simulink model "MIL4L3_SW6_V1_20220211"  (R2018b)
settings: Solver=FixedStepAuto  StartTime=0.0  StopTime=inf  FixedStep=0.001  RelTol=1e-3
PreLoadFcn:
  | A0_MILtest;
undefined symbols (not defined in the file or in its folder): Clb_ICADirect_LaneDisp_StateFive, Clb_ICADirect_LaneDisp_StateFour, Clb_ICADirect_LaneDisp_StateOne, Clb_ICADirect_LaneDisp_StateThree, Clb_ICADirect_LaneDisp_StateTwo, Clb_ICADirect_LaneDisp_StateZero, Clb_ICADirect_LaneDispSW, Clb_ICADirect_TrnLghtsCom_Switch, Clb_ICADirect_TrnLghtsCom_Value, Clb_ICADirect_TrnLghtsCrtl_Inhb, IMAP_Clb_ACU_Driver_Belt, IMAP_Clb_ACU_Driver_Belt_Over, IMAP_Clb_ACU_Passenger_Belt, IMAP_Clb_ACU_Passenger_Belt_Over, IMAP_Clb_ACU_RearLeft_Belt, IMAP_Clb_ACU_RearLeft_Belt_Over, IMAP_Clb_ACU_RearMiddle_Belt, IMAP_Clb_ACU_RearMiddle_Belt_Over, IMAP_Clb_ACU_RearRight_Belt, IMAP_Clb_ACU_RearRight_Belt_Over, IMAP_Clb_AEB_Switch, IMAP_Clb_AEB_Switch_Over, IMAP_Clb_ALC_TLC_Mode, IMAP_Clb_ALC_TLC_Mode_Over, IMAP_Clb_BCM_Battery_Voltage, IMAP_Clb_BCM_Battery_Voltage_Over, IMAP_Clb_BCM_BrakeLamp_State, IMAP_Clb_BCM_BrakeLamp_State_Over, IMAP_Clb_BCM_CHMSL_Status, IMAP_Clb_BCM_CHMSL_Status_Over, IMAP_Clb_BCM_Door_Lock_State, IMAP_Clb_BCM_Door_Lock_State_Over, IMAP_Clb_BCM_FrontWiper_State, IMAP_Clb_BCM_FrontWiper_State_Over, IMAP_Clb_BCM_FrontWiper_Switch, IMAP_Clb_BCM_FrontWiper_Switch_Over, IMAP_Clb_BCM_HazardLamp, IMAP_Clb_BCM_HazardLamp_Over, IMAP_Clb_BCM_HazardLamp_Switch, IMAP_Clb_BCM_HazardLamp_Switch_Over, IMAP_Clb_BCM_HighBeam_State, IMAP_Clb_BCM_HighBeam_State_Over, IMAP_Clb_BCM_Ignition_State, IMAP_Clb_BCM_Ignition_State_Over, IMAP_Clb_BCM_IHBC_Enabled, IMAP_Clb_BCM_IHBC_Enabled_Over, IMAP_Clb_BCM_Left_Light, IMAP_Clb_BCM_Left_Light_Over, IMAP_Clb_BCM_LeftTurn_Switch, IMAP_Clb_BCM_LeftTurn_Switch_Over, IMAP_Clb_BCM_LF_Door_State, IMAP_Clb_BCM_LF_Door_State_Over, IMAP_Clb_BCM_LowBeam_State, IMAP_Clb_BCM_LowBeam_State_Over, IMAP_Clb_BCM_LR_Door_State, IMAP_Clb_BCM_LR_Door_State_Over, IMAP_Clb_BCM_RF_Door_State, IMAP_Clb_BCM_RF_Door_State_Over, IMAP_Clb_BCM_Right_Light, IMAP_Clb_BCM_Right_Light_Over ... (+547)
libraries: CarMaker4SL x2153, simulink x292, dspstat3 x3, canmsglib x2, simulink_extras x1
(part 10 of 52)

== system MIL4L3_SW6_V1_20220211/CarMaker/VehicleControl/Function/ICA ==
  note: ICAB
  note: 状态机
  note: ICA模式：
      | 0 Unactive，1 LF，2 LF(SingleLane)，3 VF，4 LC
  note: ICA状态：
      | 0 sysOFF，1 inhibit，2 ready，3 normal，4 degradation
      | 5 fault，6 active，7 sysON，8 systoON
  Bus Selector2 : BusSelector  OutputSignals=IMAPve_g_EPS_SW_Trq,IMAPve_d_EPS_Trq_State,IMAPve_d_SAS_Clb_State,IMAPve_d_SAS_Trim_State,IMAPve_d_EPS_TrqLim_State,IMAPve_g_ESC_LatAcc,IMAPve_d_ESC_LatAcc_Valid,IMAPve_g_ESC_YawRate,IMAPve_d_ESC_YawRate_Valid,IMAPve_g_ESC_VehSpd,IMAPve_g_ESC_LonAcc,IMAPve_d_ESC_LonAcc_Valid,IMAPve_g_ESC_DySlope_Accuracy,IMAPve_g_ESC_DySlope,IMAPve_g_SW_Angle,IMAPve_g_SW_Angle_Speed,IMAPve_d_BCM_HazardLamp,IMAPve_d_BCM_Left_Light,IMAPve_d_BCM_Right_Light,IMAPve_d_BCM_Opening_State,IMAPve_d_SCC_Left_SwitchSig,IMAPve_g_EMS_RealPedal,IMAPve_d_EMS_AccPedal_Fault,IMAPve_d_ESC_Veh_Standstill,IMAPve_d_TCU_Actual_Gear,IMAPve_d_ACU_Driver_Belt,IMAPve_d_SWS_Failure_Status,IMAPve_d_ESC_ESC_Active,IMAPve_d_ESC_TCS_Active,IMAPve_d_ESC_VehSpd_Valid,IMAPve_d_ESC_ABS_Active,IMAPve_d_TCU_Select_ATMode,IMAPve_d_BCM_FrontWiper_State,IMAPve_d_ACU_Passenger_Belt,IMAPve_d_EMS_Brake_Pedal,IMAPve_d_BCM_LowBeam_State,IMAPve_d_BCM_HighBeam_State,IMAPve_d_EPS_Steer_Hold_State,IMAPve_d_EPS_Warning_State,IMAPve_d_ESC_AVH_Status,IMAPve_g_ORI_L0_C3,IMAPve_g_ORI_L0_C2,IMAPve_g_ORI_L0_C1,IMAPve_g_ORI_L0_C0,IMAPve_d_ORI_L0_Type,IMAPve_g_ORI_L0_VR,IMAPve_g_ORI_L0_W,IMAPve_g_ORI_L1_C3,IMAPve_g_ORI_L1_C2,IMAPve_g_ORI_L1_C1,IMAPve_g_ORI_L1_C0,IMAPve_d_ORI_L1_Type,IMAPve_g_ORI_L1_VR,IMAPve_g_ORI_L1_W,IMAPve_g_ORI_R0_C3,IMAPve_g_ORI_R0_C2,IMAPve_g_ORI_R0_C1,IMAPve_g_ORI_R0_C0,IMAPve_d_ORI_R0_LT,IMAPve_g_ORI_R0_VR,IMAPve_g_ORI_R0_W,IMAPve_g_ORI_R1_C3,IMAPve_g_ORI_R1_C2,IMAPve_g_ORI_R1_C1,IMAPve_g_ORI_R1_C0,IMAPve_d_ORI_R1_LT,IMAPve_g_ORI_R1_VR,IMAPve_g_ORI_R1_W,IMAPve_d_Fusion_Status,IMAPve_d_obj_Num,IMAPva_d_obj_id,IMAPva_g_obj_pos_x,IMAPva_g_obj_pos_y,IMAPva_g_obj_vel_x,IMAPva_g_obj_vel_y,IMAPva_g_obj_acc_x,IMAPva_g_obj_acc_y,IMAPva_g_obj_pos_var_x,IMAPva_g_obj_pos_var_y,IMAPva_g_obj_pos_var_xy,IMAPva_g_obj_width,IMAPva_g_obj_length,IMAPva_d_obj_class,IMAPva_d_obj_lane,IMAPva_d_obj_status,IMAPva_d_obj_age,IMAPva_d_obj_TurnLight,IMAPva_d_obj_BrakeLight,IMAPva_d_obj_MotionStatus,IMAPve_d_Road_Type,IMAPve_g_L0_C0,IMAPve_g_L0_C1,IMAPve_g_L0_C2,IMAPve_g_L0_C3,IMAPve_g_L0_VR,IMAPve_d_L0_Q,IMAPve_d_L0_Type,IMAPve_g_L0_W,IMAPve_g_R0_C0,IMAPve_g_R0_C1,IMAPve_g_R0_C2,IMAPve_g_R0_C3,IMAPve_g_R0_VR,IMAPve_d_R0_Q,IMAPve_d_R0_Type,IMAPve_g_R0_W,IMAPve_g_L1_C0,IMAPve_g_L1_C1,IMAPve_g_L1_C2,IMAPve_g_L1_C3,IMAPve_g_L1_VR,IMAPve_d_L1_Q,IMAPve_d_L1_Type,IMAPve_g_L1_W,IMAPve_g_R1_C0,IMAPve_g_R1_C1,IMAPve_g_R1_C2,IMAPve_g_R1_C3,IMAPve_g_R1_VR,IMAPve_d_R1_Q,IMAPve_d_R1_Type,IMAPve_g_R1_W,IMAPve_g_L0_C0_Back,IMAPve_g_L0_C1_Back,IMAPve_g_L0_C2_Back,IMAPve_g_L0_C3_Back,IMAPve_g_L0_Range_Back,IMAPve_g_R0_C0_Back,IMAPve_g_R0_C1_Back,IMAPve_g_R0_C2_Back,IMAPve_g_R0_C3_Back,IMAPve_g_R0_Range_Back,IMAPve_g_L1_C0_Back,IMAPve_g_L1_C1_Back,IMAPve_g_L1_C2_Back,IMAPve_g_L1_C3_Back,IMAPve_g_L1_Range_Back,IMAPve_g_R1_C0_Back,IMAPve_g_R1_C1_Back,IMAPve_g_R1_C2_Back,IMAPve_g_R1_C3_Back,IMAPve_g_R1_Range_Back,IMAPve_d_APA_AutoPark_WorkSt
  Bus Selector3 : BusSelector  OutputSignals=IMAPve_d_BCM_HazardLamp_Switch,IMAPve_d_BCM_LeftTurn_Switch,IMAPve_d_BCM_RightTurn_Switch,IMAPve_g_Lrg_C0_BACK,IMAPve_g_Lrg_C1_BACK,IMAPve_g_Lrg_C2_BACK,IMAPve_g_Lrg_C3_BACK,IMAPve_g_Lrg_VR_Start_BACK,IMAPve_g_Lrg_VR_End_BACK,IMAPve_d_Lrg_Q_BACK,IMAPve_d_Lrg_TYPE_BACK,IMAPve_g_Rrg_C0_BACK,IMAPve_g_Rrg_C1_BACK,IMAPve_g_Rrg_C2_BACK,IMAPve_g_Rrg_C3_BACK,IMAPve_g_Rrg_VR_Start_BACK,IMAPve_g_Rrg_VR_End_BACK,IMAPve_d_Rrg_Q_BACK,IMAPve_d_Rrg_TYPE_BACK
  Bus Selector : BusSelector  OutputSignals=FDMMve_d_IcaFcnConf,FDMMve_d_SignalTStamp
  Bus Selector1 : BusSelector  OutputSignals=ICABve_d_ICAMode
  BusCreator : BusCreator  Inputs=16
  Clock : Clock
  Compare To Constant : simulink/Logic and Bit Operations/Compare To Constant  relop===  const=4  OutDataTypeStr=boolean
  Constant : Constant  Value=0  OutDataTypeStr=uint32
  Constant1 : Constant  Value=0  OutDataTypeStr=uint32
  Constant2 : Constant  Value=0  OutDataTypeStr=uint16
  Constant3 : Constant  OutDataTypeStr=uint8
  Constant4 : Constant  Value=0  OutDataTypeStr=uint8
  Constant5 : Constant  OutDataTypeStr=uint8
  Constant6 : Constant  Value=0  OutDataTypeStr=uint8
  Data Type  Conversion : DataTypeConversion
  Data Type  Conversion1 : DataTypeConversion
  Data Type Conversion{,3..7,45,94,115..116} (10 alike) : DataTypeConversion
  Data Type Conversion1 : DataTypeConversion  OutDataTypeStr=uint16
  Data Type Conversion2 : DataTypeConversion  OutDataTypeStr=uint16
  Define CM Dict : CarMaker4SL/Define CM Dict  xname=User.IO.Out.VR_RR  xmono=off  xtype=Double4  xdvaplace=IO_Out  xnstates=0  xfirststate=0  xinitial=50
  Define CM Dict1 : CarMaker4SL/Define CM Dict  xname=User.IO.In.LineChangeFlag  xmono=off  xtype=Double4  xdvaplace=VC  xnstates=0  xfirststate=0  xinitial=0
  Define CM Dict2 : CarMaker4SL/Define CM Dict  xname=User.IO.In.ICABState  xmono=off  xtype=Double4  xdvaplace=VC  xnstates=0  xfirststate=0  xinitial=0
  Define CM Dict26 : CarMaker4SL/Define CM Dict  xname=User.IO.In.ICABve_g_SteerAngleCmd  xmono=off  xtype=Double4  xdvaplace=VC  xnstates=0  xfirststate=0  xinitial=0
  Define CM Dict3 : CarMaker4SL/Define CM Dict  xname=User.IO.Out.VR_R  xmono=off  xtype=Double4  xdvaplace=IO_Out  xnstates=0  xfirststate=0  xinitial=50
  Define CM Dict4 : CarMaker4SL/Define CM Dict  xname=User.IO.Out.VR_LL  xmono=off  xtype=Double4  xdvaplace=IO_Out  xnstates=0  xfirststate=0  xinitial=50
  Define CM Dict5 : CarMaker4SL/Define CM Dict  xname=User.IO.Out.VR_L  xmono=off  xtype=Double4  xdvaplace=IO_Out  xnstates=0  xfirststate=0  xinitial=50
  Define CM Dict6 : CarMaker4SL/Define CM Dict  xname=User.IO.Out.stLCRMode  xmono=off  xtype=Double4  xdvaplace=IO_Out  xnstates=0  xfirststate=0  xinitial=0
  Demux : Demux  Outputs=20
  EPS Position Control Enable Management (EPSPCEM)_KDK1 : Subsystem
  EPS_State_Mashine : Subsystem
  Enabled Subsystem : Subsystem  TreatAsAtomicUnit=on
  Goto1 : Goto  Commented=on  GotoTag=ICAS_output  TagVisibility=global
  ICAB : ModelReference  ModelNameDialog=ICAB_V51_G59_SW6_0127_MIL.slxp  ModelReferenceVersion=1.2185  CopyOfModelProtected=on
  Memory : Memory
  Read CM Dict : CarMaker4SL/Read CM Dict  xname=User.IO.Out.VR_RR  xsync=off
  Read CM Dict1 : CarMaker4SL/Read CM Dict  xname=User.IO.Out.VR_R  xsync=off
  Read CM Dict2 : CarMaker4SL/Read CM Dict  xname=User.IO.Out.VR_LL  xsync=off
  Read CM Dict3 : CarMaker4SL/Read CM Dict  xname=User.IO.Out.VR_L  xsync=off
  Switch{,1..3} (4 alike) : Switch  Threshold=20
  Write CM Dict : CarMaker4SL/Write CM Dict  xname=User.IO.Out.stLCRMode  xsync=off
  Write CM Dict1 : CarMaker4SL/Write CM Dict  xname=User.IO.In.LineChangeFlag  xsync=off
  Write CM Dict17 : CarMaker4SL/Write CM Dict  xname=User.IO.In.ICABve_g_SteerAngleCmd  xsync=off
  Write CM Dict2 : CarMaker4SL/Write CM Dict  xname=User.IO.In.ICABState  xsync=off
  ICAS_output : Outport
  tag scope: EPS_LKA_State_ica=global, ICAB_output=global, ICABva_d_ICAB2ACCS=global, ICABve_d_ICAState=global, ICAMode=global
  wires:
  [FDMM_output] -> Bus Selector/1  "FDMM_output"
  ICAB/2 -> BusCreator/2  "ICABve_d_SignalTStamp"
  Data Type Conversion2/1 -> [EPS_LKA_State_ica], EPS Position Control Enable Management (EPSPCEM)_KDK1/2(EPS_Ctr_State)
  EPS_State_Mashine/1(EPS_Ctr_State) -> Memory/1
  Data Type Conversion1/1 -> EPS_State_Mashine/1(EPS_CMD_KDK)
  EPS Position Control Enable Management (EPSPCEM)_KDK1/1(stEPS_State_Ctl_CMD) -> Data Type Conversion1/1  "EPS_State_Ctl"
  Bus Selector1/1 -> EPS Position Control Enable Management (EPSPCEM)_KDK1/1(EPSPCEM__bsTHState)  "<ICABve_d_ICAMode>"
  Bus Selector/1 -> Data Type Conversion/1  "<FDMMve_d_IcaFcnConf>"
  Clock/1 -> Data Type Conversion94/1
  [ACCSva_d_ACCS2ICAB] -> ICAB/2  "ACCSva_d_ACCS2ICA"
  ? -> Goto1/1, ICAS_output/1
  Data Type Conversion94/1 -> ICAB/1  "System_Clock"
  BusCreator/1 -> Bus Selector1/1, [ICAB_output]
  Data Type  Conversion/1 -> Data Type  Conversion1/1, BusCreator/4  "ICABve_g_SteerAngleCmd"
  Data Type Conversion116/1 -> Write CM Dict2/1
  [IMAP_Output] -> Bus Selector3/1, Bus Selector2/1  "FDMM_output"
  [EPS_LKA_State_ica] -> ICAB/5
  ICAB/16 -> BusCreator/16  "ICABve_g_ob011L_100"
  ICAB/15 -> BusCreator/15  "ICABve_g_ob011H_100"
  ICAB/14 -> BusCreator/14  "ICABve_g_ob010L_100"
  ICAB/13 -> BusCreator/13  "ICABve_g_ob010H_100"
  ICAB/12 -> BusCreator/12  "ICABve_g_ob8L_10"
  ICAB/11 -> BusCreator/11  "ICABve_g_ob8H_10"
  Bus Selector/2 -> ICAB/4  "<FDMMve_d_SignalTStamp>"
  Data Type  Conversion1/1 -> Write CM Dict17/1  "ICABve_g_SteerAngleCmd"
  Data Type Conversion45/1 -> Write CM Dict1/1
  Enabled Subsystem/1(Out1) -> Data Type Conversion45/1
  Compare To Constant/1 -> Enabled Subsystem/Enable
  ICAB/1 -> [ICABva_d_ICAB2ACCS], BusCreator/1  "ICABva_d_ICAB2ACCS"
  ICAB/4 -> Data Type  Conversion/1
  Data Type Conversion115/1 -> [ICAMode], BusCreator/5  "ICABve_d_ICAMode"
  ICAB/6 -> [ICABve_d_ICAState], BusCreator/6, Data Type Conversion116/1  "ICABve_d_ICAState"
  ICAB/7 -> BusCreator/7  "ICABve_d_LKATorqueReq"
  ICAB/8 -> BusCreator/8  "ICABve_g_LKATorqueReq_Value"
  ICAB/9 -> BusCreator/9  "ICABve_g_ob7H_10"
  ICAB/10 -> BusCreator/10  "ICABve_g_ob7L_10"
  Demux/16 -> Data Type Conversion7/1
  ICAB/3 -> BusCreator/3, Demux/1  "ICABva_d_ICAB2HMI"
  Data Type Conversion7/1 -> Write CM Dict/1  "stLCRMode"
  Memory/1 -> Data Type Conversion2/1
  Data Type Conversion/1 -> ICAB/3
  Bus Selector2/118 -> ICAB/123  "<IMAPve_g_R1_C3>"
  Bus Selector2/120 -> ICAB/125  "<IMAPve_d_R1_Q>"
  Bus Selector2/117 -> ICAB/122  "<IMAPve_g_R1_C2>"
  Bus Selector2/121 -> ICAB/126  "<IMAPve_d_R1_Type>"
  Bus Selector2/116 -> ICAB/121  "<IMAPve_g_R1_C1>"
  Bus Selector2/122 -> ICAB/127  "<IMAPve_g_R1_W>"
  Bus Selector2/115 -> ICAB/120  "<IMAPve_g_R1_C0>"
  Bus Selector2/123 -> ICAB/128  "<IMAPve_g_L0_C0_Back>"
  Bus Selector2/114 -> ICAB/119  "<IMAPve_g_L1_W>"
  Bus Selector2/124 -> ICAB/129  "<IMAPve_g_L0_C1_Back>"
  Bus Selector2/113 -> ICAB/118  "<IMAPve_d_L1_Type>"
  Bus Selector2/125 -> ICAB/130  "<IMAPve_g_L0_C2_Back>"
  Bus Selector2/112 -> ICAB/117  "<IMAPve_d_L1_Q>"
  Bus Selector2/126 -> ICAB/131  "<IMAPve_g_L0_C3_Back>"
  Bus Selector2/127 -> ICAB/132  "<IMAPve_g_L0_Range_Back>"
  Bus Selector2/110 -> ICAB/115  "<IMAPve_g_L1_C3>"
  Bus Selector2/128 -> ICAB/133  "<IMAPve_g_R0_C0_Back>"
  Bus Selector2/109 -> ICAB/114  "<IMAPve_g_L1_C2>"
  Bus Selector2/129 -> ICAB/134  "<IMAPve_g_R0_C1_Back>"
  Bus Selector2/108 -> ICAB/113  "<IMAPve_g_L1_C1>"
  Bus Selector2/130 -> ICAB/135  "<IMAPve_g_R0_C2_Back>"
  Bus Selector2/107 -> ICAB/112  "<IMAPve_g_L1_C0>"
  Bus Selector2/131 -> ICAB/136  "<IMAPve_g_R0_C3_Back>"
  Bus Selector2/106 -> ICAB/111  "<IMAPve_g_R0_W>"
  Bus Selector2/132 -> ICAB/137  "<IMAPve_g_R0_Range_Back>"
  Bus Selector2/105 -> ICAB/110  "<IMAPve_d_R0_Type>"
  Bus Selector2/133 -> ICAB/138  "<IMAPve_g_L1_C0_Back>"
  Bus Selector2/104 -> ICAB/109  "<IMAPve_d_R0_Q>"
  Bus Selector2/134 -> ICAB/139  "<IMAPve_g_L1_C1_Back>"
  Bus Selector2/135 -> ICAB/140  "<IMAPve_g_L1_C2_Back>"
  Bus Selector2/102 -> ICAB/107  "<IMAPve_g_R0_C3>"
  Bus Selector2/136 -> ICAB/141  "<IMAPve_g_L1_C3_Back>"
  Bus Selector2/101 -> ICAB/106  "<IMAPve_g_R0_C2>"
  Bus Selector2/137 -> ICAB/142  "<IMAPve_g_L1_Range_Back>"
  Bus Selector2/100 -> ICAB/105  "<IMAPve_g_R0_C1>"
  Bus Selector2/138 -> ICAB/143  "<IMAPve_g_R1_C0_Back>"
  Bus Selector2/99 -> ICAB/104  "<IMAPve_g_R0_C0>"
  Bus Selector2/139 -> ICAB/144  "<IMAPve_g_R1_C1_Back>"
  Bus Selector2/98 -> ICAB/103  "<IMAPve_g_L0_W>"
  Bus Selector2/140 -> ICAB/145  "<IMAPve_g_R1_C2_Back>"
  Bus Selector2/97 -> ICAB/102  "<IMAPve_d_L0_Type>"
  Bus Selector2/141 -> ICAB/146  "<IMAPve_g_R1_C3_Back>"
  Bus Selector2/96 -> ICAB/101  "<IMAPve_d_L0_Q>"
  Bus Selector2/142 -> ICAB/147  "<IMAPve_g_R1_Range_Back>"
  Switch3/1 -> ICAB/100
  Bus Selector2/143 -> ICAB/148  "<IMAPve_d_APA_AutoPark_WorkSt>"
  Bus Selector2/94 -> ICAB/99  "<IMAPve_g_L0_C3>"
  Bus Selector2/93 -> ICAB/98  "<IMAPve_g_L0_C2>"
  Bus Selector2/92 -> ICAB/97  "<IMAPve_g_L0_C1>"
  Bus Selector2/91 -> ICAB/96  "<IMAPve_g_L0_C0>"
  Bus Selector2/90 -> ICAB/95  "<IMAPve_d_Road_Type>"
  Bus Selector2/89 -> ICAB/94  "<IMAPva_d_obj_MotionStatus>"
  Bus Selector2/88 -> ICAB/93  "<IMAPva_d_obj_BrakeLight>"
  Bus Selector2/87 -> ICAB/92  "<IMAPva_d_obj_TurnLight>"
  Bus Selector2/86 -> ICAB/91  "<IMAPva_d_obj_age>"
  Bus Selector2/85 -> ICAB/90  "<IMAPva_d_obj_status>"
  Bus Selector2/84 -> ICAB/89  "<IMAPva_d_obj_lane>"
  Bus Selector2/83 -> ICAB/88  "<IMAPva_d_obj_class>"
  Bus Selector2/82 -> ICAB/87  "<IMAPva_g_obj_length>"
  Bus Selector2/81 -> ICAB/86  "<IMAPva_g_obj_width>"
  Bus Selector2/80 -> ICAB/85  "<IMAPva_g_obj_pos_var_xy>"
  Bus Selector2/79 -> ICAB/84  "<IMAPva_g_obj_pos_var_y>"
  Bus Selector2/78 -> ICAB/83  "<IMAPva_g_obj_pos_var_x>"
  Bus Selector2/77 -> ICAB/82  "<IMAPva_g_obj_acc_y>"
  Bus Selector2/76 -> ICAB/81  "<IMAPva_g_obj_acc_x>"
  Bus Selector2/75 -> ICAB/80  "<IMAPva_g_obj_vel_y>"
  Bus Selector2/74 -> ICAB/79  "<IMAPva_g_obj_vel_x>"
  Bus Selector2/73 -> ICAB/78  "<IMAPva_g_obj_pos_y>"
  Bus Selector2/72 -> ICAB/77  "<IMAPva_g_obj_pos_x>"
  Bus Selector2/71 -> ICAB/76  "<IMAPva_d_obj_id>"
  Bus Selector2/70 -> ICAB/75  "<IMAPve_d_obj_Num>"
  Bus Selector2/69 -> ICAB/74  "<IMAPve_d_Fusion_Status>"
  Bus Selector2/68 -> ICAB/73  "<IMAPve_g_ORI_R1_W>"
  Bus Selector2/67 -> ICAB/72  "<IMAPve_g_ORI_R1_VR>"
  Bus Selector2/66 -> ICAB/71  "<IMAPve_d_ORI_R1_LT>"
  Bus Selector2/65 -> ICAB/70  "<IMAPve_g_ORI_R1_C0>"
  Bus Selector2/64 -> ICAB/69  "<IMAPve_g_ORI_R1_C1>"
  Bus Selector2/63 -> ICAB/68  "<IMAPve_g_ORI_R1_C2>"
  Bus Selector2/62 -> ICAB/67  "<IMAPve_g_ORI_R1_C3>"
  Bus Selector2/61 -> ICAB/66  "<IMAPve_g_ORI_R0_W>"
  Bus Selector2/60 -> ICAB/65  "<IMAPve_g_ORI_R0_VR>"
  Bus Selector2/59 -> ICAB/64  "<IMAPve_d_ORI_R0_LT>"
  Bus Selector2/58 -> ICAB/63  "<IMAPve_g_ORI_R0_C0>"
  Bus Selector2/57 -> ICAB/62  "<IMAPve_g_ORI_R0_C1>"
  Bus Selector2/56 -> ICAB/61  "<IMAPve_g_ORI_R0_C2>"
  Bus Selector2/55 -> ICAB/60  "<IMAPve_g_ORI_R0_C3>"
  Bus Selector2/54 -> ICAB/59  "<IMAPve_g_ORI_L1_W>"
  Bus Selector2/53 -> ICAB/58  "<IMAPve_g_ORI_L1_VR>"
  Bus Selector2/52 -> ICAB/57  "<IMAPve_d_ORI_L1_Type>"
  Bus Selector2/51 -> ICAB/56  "<IMAPve_g_ORI_L1_C0>"
  Bus Selector2/50 -> ICAB/55  "<IMAPve_g_ORI_L1_C1>"
  Bus Selector2/49 -> ICAB/54  "<IMAPve_g_ORI_L1_C2>"
  Bus Selector2/48 -> ICAB/53  "<IMAPve_g_ORI_L1_C3>"
  Bus Selector2/47 -> ICAB/52  "<IMAPve_g_ORI_L0_W>"
  Bus Selector2/46 -> ICAB/51  "<IMAPve_g_ORI_L0_VR>"
  Bus Selector2/45 -> ICAB/50  "<IMAPve_d_ORI_L0_Type>"
  Bus Selector2/44 -> ICAB/49  "<IMAPve_g_ORI_L0_C0>"
  Bus Selector2/43 -> ICAB/48  "<IMAPve_g_ORI_L0_C1>"
  Bus Selector2/42 -> ICAB/47  "<IMAPve_g_ORI_L0_C2>"
  Bus Selector2/41 -> ICAB/46  "<IMAPve_g_ORI_L0_C3>"
  Bus Selector2/40 -> ICAB/45  "<IMAPve_d_ESC_AVH_Status>"
  Bus Selector2/39 -> ICAB/44  "<IMAPve_d_EPS_Warning_State>"
  Bus Selector2/38 -> ICAB/43  "<IMAPve_d_EPS_Steer_Hold_State>"
  Bus Selector2/37 -> ICAB/42  "<IMAPve_d_BCM_HighBeam_State>"
  Bus Selector2/36 -> ICAB/41  "<IMAPve_d_BCM_LowBeam_State>"
  Bus Selector2/35 -> ICAB/40  "<IMAPve_d_EMS_Brake_Pedal>"
  Bus Selector2/34 -> ICAB/39  "<IMAPve_d_ACU_Passenger_Belt>"
  Bus Selector2/33 -> ICAB/38  "<IMAPve_d_BCM_FrontWiper_State>"
  Bus Selector2/32 -> ICAB/37  "<IMAPve_d_TCU_Select_ATMode>"
  Bus Selector2/31 -> ICAB/36  "<IMAPve_d_ESC_ABS_Active>"
  Bus Selector2/30 -> ICAB/35  "<IMAPve_d_ESC_VehSpd_Valid>"
  Bus Selector2/29 -> ICAB/34  "<IMAPve_d_ESC_TCS_Active>"
  Bus Selector2/28 -> ICAB/33  "<IMAPve_d_ESC_ESC_Active>"
  Bus Selector2/27 -> ICAB/32  "<IMAPve_d_SWS_Failure_Status>"
  Bus Selector2/26 -> ICAB/31  "<IMAPve_d_ACU_Driver_Belt>"
  Bus Selector2/25 -> ICAB/30  "<IMAPve_d_TCU_Actual_Gear>"
  Bus Selector2/24 -> ICAB/29  "<IMAPve_d_ESC_Veh_Standstill>"
  Bus Selector2/23 -> ICAB/28  "<IMAPve_d_EMS_AccPedal_Fault>"
  Bus Selector2/22 -> ICAB/27  "<IMAPve_g_EMS_RealPedal>"
  Bus Selector2/21 -> ICAB/26  "<IMAPve_d_SCC_Left_SwitchSig>"
  Bus Selector2/20 -> ICAB/25  "<IMAPve_d_BCM_Opening_State>"
  Bus Selector2/19 -> ICAB/24  "<IMAPve_d_BCM_Right_Light>"
  Bus Selector2/18 -> ICAB/23  "<IMAPve_d_BCM_Left_Light>"
  Bus Selector2/17 -> ICAB/22  "<IMAPve_d_BCM_HazardLamp>"
  Bus Selector2/16 -> ICAB/21  "<IMAPve_g_SW_Angle_Speed>"
  Bus Selector2/15 -> ICAB/20  "<IMAPve_g_SW_Angle>"
  Bus Selector2/14 -> ICAB/19  "<IMAPve_g_ESC_DySlope>"
  Bus Selector2/13 -> ICAB/18  "<IMAPve_g_ESC_DySlope_Accuracy>"
  Bus Selector2/12 -> ICAB/17  "<IMAPve_d_ESC_LonAcc_Valid>"
  Bus Selector2/11 -> ICAB/16  "<IMAPve_g_ESC_LonAcc>"
  Bus Selector2/10 -> ICAB/15  "<IMAPve_g_ESC_VehSpd>"
  Bus Selector2/9 -> ICAB/14  "<IMAPve_d_ESC_YawRate_Valid>"
  Bus Selector2/8 -> ICAB/13  "<IMAPve_g_ESC_YawRate>"
  Bus Selector2/7 -> ICAB/12  "<IMAPve_d_ESC_LatAcc_Valid>"
  Bus Selector2/6 -> ICAB/11  "<IMAPve_g_ESC_LatAcc>"
  Bus Selector2/5 -> ICAB/10  "<IMAPve_d_EPS_TrqLim_State>"
  Bus Selector2/4 -> ICAB/9  "<IMAPve_d_SAS_Trim_State>"
  Bus Selector2/3 -> ICAB/8  "<IMAPve_d_SAS_Clb_State>"
  Bus Selector2/2 -> ICAB/7  "<IMAPve_d_EPS_Trq_State>"
  Bus Selector2/1 -> ICAB/6  "<IMAPve_g_EPS_SW_Trq>"
  Bus Selector3/1 -> ICAB/156  "<IMAPve_d_BCM_HazardLamp_Switch>"
  Bus Selector3/2 -> ICAB/157  "<IMAPve_d_BCM_LeftTurn_Switch>"
  Bus Selector3/3 -> ICAB/158  "<IMAPve_d_BCM_RightTurn_Switch>"
  Bus Selector3/4 -> ICAB/159  "<IMAPve_g_Lrg_C0_BACK>"
  Bus Selector3/5 -> ICAB/160  "<IMAPve_g_Lrg_C1_BACK>"
  Bus Selector3/6 -> ICAB/161  "<IMAPve_g_Lrg_C2_BACK>"
  Bus Selector3/7 -> ICAB/162  "<IMAPve_g_Lrg_C3_BACK>"
  Bus Selector3/8 -> ICAB/163  "<IMAPve_g_Lrg_VR_Start_BACK>"
  Bus Selector3/9 -> ICAB/164  "<IMAPve_g_Lrg_VR_End_BACK>"
  Bus Selector3/10 -> ICAB/165  "<IMAPve_d_Lrg_Q_BACK>"
  Bus Selector3/11 -> ICAB/166  "<IMAPve_d_Lrg_TYPE_BACK>"
  Bus Selector3/12 -> ICAB/167  "<IMAPve_g_Rrg_C0_BACK>"
  Bus Selector3/13 -> ICAB/168  "<IMAPve_g_Rrg_C1_BACK>"
  Bus Selector3/14 -> ICAB/169  "<IMAPve_g_Rrg_C2_BACK>"
  Bus Selector3/15 -> ICAB/170  "<IMAPve_g_Rrg_C3_BACK>"
  Bus Selector3/16 -> ICAB/171  "<IMAPve_g_Rrg_VR_Start_BACK>"
  Bus Selector3/17 -> ICAB/172  "<IMAPve_g_Rrg_VR_End_BACK>"
  Bus Selector3/18 -> ICAB/173  "<IMAPve_d_Rrg_Q_BACK>"
  Bus Selector3/19 -> ICAB/174  "<IMAPve_d_Rrg_TYPE_BACK>"
  Constant/1 -> ICAB/149
  Constant1/1 -> ICAB/150
  Constant3/1 -> ICAB/152
  Constant5/1 -> ICAB/154
  Constant2/1 -> ICAB/151
  Constant4/1 -> ICAB/153
  Constant6/1 -> ICAB/155
  Read CM Dict3/1 -> Data Type Conversion3/1
  Data Type Conversion3/1 -> Switch3/3, Switch3/2
  Bus Selector2/95 -> Switch3/1  "<IMAPve_g_L0_VR>"
  Data Type Conversion4/1 -> Switch1/3, Switch1/2
  Read CM Dict1/1 -> Data Type Conversion4/1
  Switch1/1 -> ICAB/108  "IMAPve_g_R0_VR"
  Bus Selector2/103 -> Switch1/1  "<IMAPve_g_R0_VR>"
  Data Type Conversion5/1 -> Switch2/3, Switch2/2
  Read CM Dict2/1 -> Data Type Conversion5/1
  Switch2/1 -> ICAB/116
  Bus Selector2/111 -> Switch2/1  "<IMAPve_g_L1_VR>"
  Read CM Dict/1 -> Data Type Conversion6/1
  Data Type Conversion6/1 -> Switch/3, Switch/2
  Switch/1 -> ICAB/124  "IMAPve_g_R1_VR"
  Bus Selector2/119 -> Switch/1  "<IMAPve_g_R1_VR>"
  ICAB/5 -> Data Type Conversion115/1, Compare To Constant/1, Enabled Subsystem/1(In)  "ICABve_d_ICAMode"

== system MIL4L3_SW6_V1_20220211/CarMaker/VehicleControl/Function/ICA_ALC ==
  note: ICA状态：
      | 0 sysOFF，1 inhibit，2 ready，3 normal，4 degradation
      | 5 fault，6 active，7 sysON，8 systoON
  note: ICA模式：
      | 0 Unactive，1 LF，2 LF(SingleLane)，3 VF，4 LC
  note: 状态机
  note: ICAB
  Bus Selector2 : BusSelector  OutputSignals=IMAPve_d_RCTA_Swtich,IMAPve_d_DOW_Switch,IMAPve_d_JA_Brake_Switch,IMAPve_d_JA_Alert_Switch,IMAPve_d_EPS_LKA_State,IMAPve_d_EPS_Trq_State,IMAPve_d_SAS_Clb_State,IMAPve_d_SAS_Trim_State,IMAPve_d_EPS_TrqLim_State,IMAPve_g_ESC_LatAcc,IMAPve_d_ESC_LatAcc_Valid,IMAPve_g_ESC_YawRate,IMAPve_g_ESC_VehSpd,IMAPve_g_ESC_LonAcc,IMAPve_d_ESC_LonAcc_Valid,IMAPve_g_ESC_Brake_Press,IMAPve_g_ESC_Static_Slope,IMAPve_g_ESC_DySlope_Accuracy,IMAPve_g_ESC_DySlope,IMAPve_g_SW_Angle_Speed,IMAPve_d_BCM_Trunk_State,IMAPve_d_PEPS_Door_Lock_Req,IMAPve_g_EMS_MinTWhl_Offset,IMAPve_g_EMS_ACC_VirtualPedal,IMAPve_d_EMS_AccPedal_Fault,IMAPve_d_ESC_Veh_Standstill,IMAPve_d_TCU_Actual_Gear,IMAPve_d_BCM_Ignition_State,IMAPve_d_SWS_Failure_Status,IMAPve_d_ESC_OFF,IMAPve_d_ESC_AlarmSig,IMAPve_d_ESC_RR_Wheel_Pulse,IMAPve_d_ESC_AEB_Available,IMAPve_d_ESC_ACC_Active,IMAPve_d_BCM_CHMSL_Status,IMAPve_d_BCM_BrakeLamp_State,IMAPve_d_ACU_Passenger_Belt,IMAPve_d_EPB_Warn_Req,IMAPve_d_EPB_Switch_State,IMAPve_d_ESC_Hold_State,IMAPva_g_ORI_Obj_LongDis,IMAPva_g_ORI_Obj_LAngle,IMAPva_g_ORI_Obj_RAngle,IMAPva_g_ORI_Obj_Width,IMAPva_d_ORI_Obj_ID,IMAPve_g_ORI_L0_C3,IMAPve_g_ORI_L0_C2,IMAPve_g_ORI_L0_C1,IMAPve_g_ORI_L0_C0,IMAPve_d_ORI_L0_Type,IMAPve_g_ORI_L0_VR,IMAPve_g_ORI_L0_W,IMAPve_g_ORI_L1_C3,IMAPve_g_ORI_L1_C2,IMAPve_g_ORI_L1_C1,IMAPve_g_ORI_L1_C0,IMAPve_d_ORI_L1_Type,IMAPve_g_ORI_L1_VR,IMAPve_g_ORI_L1_W,IMAPve_g_ORI_R0_C3,IMAPve_g_ORI_R0_C2,IMAPve_g_ORI_R0_C1,IMAPve_g_ORI_R0_C0,IMAPve_d_ORI_R0_LT,IMAPve_g_ORI_R0_VR,IMAPve_g_ORI_R0_W,IMAPve_g_ORI_R1_C3,IMAPve_g_ORI_R1_C2,IMAPve_d_Sensor_Status,IMAPve_d_RF_Radar_Status,IMAPve_d_LR_Radar_Status,IMAPve_d_RR_Radar_Status,IMAPve_d_Fusion_Status,IMAPve_d_Fusion_Time_Stamp,IMAPve_d_obj_Num,IMAPva_d_obj_id,IMAPva_g_obj_pos_x,IMAPva_g_obj_pos_y,IMAPva_g_obj_vel_x,IMAPva_g_obj_vel_y,IMAPva_g_obj_acc_x,IMAPva_g_obj_acc_y,IMAPva_g_obj_pos_var_x,IMAPva_g_obj_pos_var_y,IMAPva_g_obj_pos_var_xy,IMAPva_g_obj_width,IMAPva_g_obj_length,IMAPva_d_obj_class,IMAPva_d_obj_lane,IMAPva_d_obj_status,IMAPva_d_obj_age,IMAPva_d_obj_TurnLight,IMAPva_d_obj_BrakeLight,IMAPva_d_obj_MotionStatus,IMAPve_d_Road_Type,IMAPve_g_L0_C0,IMAPve_g_L0_C1,IMAPve_g_L0_C2,IMAPve_g_L0_C3,IMAPve_g_L0_VR,IMAPve_d_L0_Q,IMAPve_d_L0_Type,IMAPve_g_L0_W,IMAPve_g_R0_C0,IMAPve_g_R0_C1,IMAPve_g_R0_C2,IMAPve_g_R0_C3,IMAPve_g_R0_VR,IMAPve_d_R0_Q,IMAPve_d_R0_Type,IMAPve_g_R0_W,IMAPve_g_L1_C0,IMAPve_g_L1_C1,IMAPve_g_L1_C2,IMAPve_g_L1_C3,IMAPve_g_L1_VR,IMAPve_d_L1_Q,IMAPve_d_L1_Type,IMAPve_g_L1_W,IMAPve_g_R1_C0,IMAPve_g_R1_C1,IMAPve_g_R1_C2,IMAPve_g_R1_C3,IMAPve_g_R1_VR,IMAPve_d_R1_Q,IMAPve_d_R1_Type,IMAPve_g_R1_W,IMAPve_g_L0_C0_Back,IMAPve_g_L0_C1_Back,IMAPve_g_L0_C2_Back,IMAPve_g_L0_C3_Back,IMAPve_g_L0_Range_Back,IMAPve_g_R0_C0_Back,IMAPve_g_R0_C1_Back,IMAPve_g_R0_C2_Back,IMAPve_g_R0_C3_Back,IMAPve_g_R0_Range_Back,IMAPve_g_L1_C0_Back,IMAPve_g_L1_C1_Back,IMAPve_g_L1_C2_Back,IMAPve_g_L1_C3_Back,IMAPve_g_L1_Range_Back,IMAPve_d_APA_AutoPark_WorkSt
  Bus Selector3 : BusSelector  OutputSignals=IMAPve_d_BCM_RF_Door_State,IMAPve_d_TSR_Sign_Type,IMAPve_g_Camera_Signal_Fault
  Bus Selector : BusSelector  OutputSignals=FDMMve_d_IcaFcnConf,FDMMve_d_SignalTStamp
  Bus Selector1 : BusSelector  OutputSignals=ICABve_d_ICAMode
  BusCreator : BusCreator  Inputs=18
  Clock : Clock
  Compare To Constant : simulink/Logic and Bit Operations/Compare To Constant  relop===  const=4  OutDataTypeStr=boolean
  Constant : Constant  Value=0  OutDataTypeStr=uint32
  Constant1 : Constant  Value=0  OutDataTypeStr=uint32
  Constant2 : Constant  Value=0  OutDataTypeStr=uint16
  Constant3 : Constant  OutDataTypeStr=uint8
  Constant4 : Constant  Value=0  OutDataTypeStr=uint8
  Constant5 : Constant  OutDataTypeStr=uint8
  Constant6 : Constant  Value=0  OutDataTypeStr=uint8
  Data Type  Conversion : DataTypeConversion
  Data Type  Conversion1 : DataTypeConversion
  Data Type Conversion{,3..7,45,94,115..116} (10 alike) : DataTypeConversion
  Data Type Conversion1 : DataTypeConversion  OutDataTypeStr=uint16
  Data Type Conversion2 : DataTypeConversion  OutDataTypeStr=uint16
  Define CM Dict : CarMaker4SL/Define CM Dict  xname=User.IO.Out.VR_RR  xmono=off  xtype=Double4  xdvaplace=IO_Out  xnstates=0  xfirststate=0  xinitial=50
  Define CM Dict1 : CarMaker4SL/Define CM Dict  xname=User.IO.In.LineChangeFlag  xmono=off  xtype=Double4  xdvaplace=VC  xnstates=0  xfirststate=0  xinitial=0
  Define CM Dict2 : CarMaker4SL/Define CM Dict  xname=User.IO.In.ICABState  xmono=off  xtype=Double4  xdvaplace=VC  xnstates=0  xfirststate=0  xinitial=0
  Define CM Dict26 : CarMaker4SL/Define CM Dict  xname=User.IO.In.ICABve_g_SteerAngleCmd  xmono=off  xtype=Double4  xdvaplace=VC  xnstates=0  xfirststate=0  xinitial=0
  Define CM Dict3 : CarMaker4SL/Define CM Dict  xname=User.IO.Out.VR_R  xmono=off  xtype=Double4  xdvaplace=IO_Out  xnstates=0  xfirststate=0  xinitial=50
  Define CM Dict4 : CarMaker4SL/Define CM Dict  xname=User.IO.Out.VR_LL  xmono=off  xtype=Double4  xdvaplace=IO_Out  xnstates=0  xfirststate=0  xinitial=50
  Define CM Dict5 : CarMaker4SL/Define CM Dict  xname=User.IO.Out.VR_L  xmono=off  xtype=Double4  xdvaplace=IO_Out  xnstates=0  xfirststate=0  xinitial=50
  Define CM Dict6 : CarMaker4SL/Define CM Dict  xname=User.IO.Out.stLCRMode  xmono=off  xtype=Double4  xdvaplace=IO_Out  xnstates=0  xfirststate=0  xinitial=0
  Demux : Demux  Outputs=20
  EPS Position Control Enable Management (EPSPCEM)_KDK1 : Subsystem
  EPS_State_Mashine : Subsystem
  Enabled Subsystem : Subsystem  TreatAsAtomicUnit=on
  Goto1 : Goto  Commented=on  GotoTag=ICAS_output  TagVisibility=global
  ICAB : ModelReference  ModelNameDialog=Mil_ICAB_V41_G59_SW5_1229.slxp  ModelReferenceVersion=1.1943  CopyOfModelProtected=on
  Memory : Memory
  Read CM Dict : CarMaker4SL/Read CM Dict  xname=User.IO.Out.VR_RR  xsync=off
  Read CM Dict1 : CarMaker4SL/Read CM Dict  xname=User.IO.Out.VR_R  xsync=off
  Read CM Dict2 : CarMaker4SL/Read CM Dict  xname=User.IO.Out.VR_LL  xsync=off
  Read CM Dict3 : CarMaker4SL/Read CM Dict  xname=User.IO.Out.VR_L  xsync=off
  Switch{,1..3} (4 alike) : Switch  Threshold=20
  Write CM Dict : CarMaker4SL/Write CM Dict  xname=User.IO.Out.stLCRMode  xsync=off
  Write CM Dict1 : CarMaker4SL/Write CM Dict  xname=User.IO.In.LineChangeFlag  xsync=off
  Write CM Dict17 : CarMaker4SL/Write CM Dict  xname=User.IO.In.ICABve_g_SteerAngleCmd  xsync=off
  Write CM Dict2 : CarMaker4SL/Write CM Dict  xname=User.IO.In.ICABState  xsync=off
  ICAS_output : Outport
  tag scope: EPS_LKA_State_alc=global, ICAB_output=global, ICABva_d_ICAB2ACCS=global, ICABve_d_ICAState=global
  wires:
  Data Type Conversion/1 -> ICAB/3
  Bus Selector2/96 -> ICAB/101  "<IMAPve_g_L0_C0>"
  Bus Selector2/142 -> ICAB/147  "<IMAPve_g_L1_Range_Back>"
  Bus Selector2/141 -> ICAB/146  "<IMAPve_g_L1_C3_Back>"
  Bus Selector2/140 -> ICAB/145  "<IMAPve_g_L1_C2_Back>"
  Bus Selector2/139 -> ICAB/144  "<IMAPve_g_L1_C1_Back>"
  Bus Selector2/138 -> ICAB/143  "<IMAPve_g_L1_C0_Back>"
  Bus Selector2/137 -> ICAB/142  "<IMAPve_g_R0_Range_Back>"
  Bus Selector2/136 -> ICAB/141  "<IMAPve_g_R0_C3_Back>"
  Bus Selector2/135 -> ICAB/140  "<IMAPve_g_R0_C2_Back>"
  Bus Selector2/134 -> ICAB/139  "<IMAPve_g_R0_C1_Back>"
  Bus Selector2/133 -> ICAB/138  "<IMAPve_g_R0_C0_Back>"
  Bus Selector2/132 -> ICAB/137  "<IMAPve_g_L0_Range_Back>"
  Bus Selector2/131 -> ICAB/136  "<IMAPve_g_L0_C3_Back>"
  Bus Selector2/130 -> ICAB/135  "<IMAPve_g_L0_C2_Back>"
  Bus Selector2/129 -> ICAB/134  "<IMAPve_g_L0_C1_Back>"
  Bus Selector2/128 -> ICAB/133  "<IMAPve_g_L0_C0_Back>"
  Bus Selector2/127 -> ICAB/132  "<IMAPve_g_R1_W>"
  Bus Selector2/126 -> ICAB/131  "<IMAPve_d_R1_Type>"
  Bus Selector2/125 -> ICAB/130  "<IMAPve_d_R1_Q>"
  Bus Selector2/124 -> ICAB/129  "<IMAPve_g_R1_VR>"
  Bus Selector2/123 -> ICAB/128  "<IMAPve_g_R1_C3>"
  Bus Selector2/122 -> ICAB/127  "<IMAPve_g_R1_C2>"
  Bus Selector2/121 -> ICAB/126  "<IMAPve_g_R1_C1>"
  Bus Selector2/120 -> ICAB/125  "<IMAPve_g_R1_C0>"
  Bus Selector2/118 -> ICAB/123  "<IMAPve_d_L1_Type>"
  Bus Selector2/117 -> ICAB/122  "<IMAPve_d_L1_Q>"
  Bus Selector2/116 -> ICAB/121  "<IMAPve_g_L1_VR>"
  Bus Selector2/115 -> ICAB/120  "<IMAPve_g_L1_C3>"
  Bus Selector2/114 -> ICAB/119  "<IMAPve_g_L1_C2>"
  Bus Selector2/113 -> ICAB/118  "<IMAPve_g_L1_C1>"
  Bus Selector2/112 -> ICAB/117  "<IMAPve_g_L1_C0>"
  Bus Selector2/110 -> ICAB/115  "<IMAPve_d_R0_Type>"
  Bus Selector2/109 -> ICAB/114  "<IMAPve_d_R0_Q>"
  Bus Selector2/108 -> ICAB/113  "<IMAPve_g_R0_VR>"
  Bus Selector2/107 -> ICAB/112  "<IMAPve_g_R0_C3>"
  Bus Selector2/106 -> ICAB/111  "<IMAPve_g_R0_C2>"
  Bus Selector2/105 -> ICAB/110  "<IMAPve_g_R0_C1>"
  Bus Selector2/104 -> ICAB/109  "<IMAPve_g_R0_C0>"
  Bus Selector2/102 -> ICAB/107  "<IMAPve_d_L0_Type>"
  Bus Selector2/101 -> ICAB/106  "<IMAPve_d_L0_Q>"
  Bus Selector2/100 -> ICAB/105  "<IMAPve_g_L0_VR>"
  Bus Selector2/99 -> ICAB/104  "<IMAPve_g_L0_C3>"
  Bus Selector2/98 -> ICAB/103  "<IMAPve_g_L0_C2>"
  Bus Selector2/97 -> ICAB/102  "<IMAPve_g_L0_C1>"
  Bus Selector2/94 -> ICAB/99  "<IMAPva_d_obj_MotionStatus>"
  Bus Selector2/93 -> ICAB/98  "<IMAPva_d_obj_BrakeLight>"
  Bus Selector2/92 -> ICAB/97  "<IMAPva_d_obj_TurnLight>"
  Bus Selector2/91 -> ICAB/96  "<IMAPva_d_obj_age>"
  Bus Selector2/90 -> ICAB/95  "<IMAPva_d_obj_status>"
  Bus Selector2/89 -> ICAB/94  "<IMAPva_d_obj_lane>"
  Bus Selector2/88 -> ICAB/93  "<IMAPva_d_obj_class>"
  Bus Selector2/87 -> ICAB/92  "<IMAPva_g_obj_length>"
  Bus Selector2/86 -> ICAB/91  "<IMAPva_g_obj_width>"
  Bus Selector2/85 -> ICAB/90  "<IMAPva_g_obj_pos_var_xy>"
  Bus Selector2/84 -> ICAB/89  "<IMAPva_g_obj_pos_var_y>"
  Bus Selector2/83 -> ICAB/88  "<IMAPva_g_obj_pos_var_x>"
  Bus Selector2/82 -> ICAB/87  "<IMAPva_g_obj_acc_y>"
  Bus Selector2/81 -> ICAB/86  "<IMAPva_g_obj_acc_x>"
  Bus Selector2/80 -> ICAB/85  "<IMAPva_g_obj_vel_y>"
  Bus Selector2/79 -> ICAB/84  "<IMAPva_g_obj_vel_x>"
  Bus Selector2/78 -> ICAB/83  "<IMAPva_g_obj_pos_y>"
  Bus Selector2/77 -> ICAB/82  "<IMAPva_g_obj_pos_x>"
  Bus Selector2/76 -> ICAB/81  "<IMAPva_d_obj_id>"
  Bus Selector2/75 -> ICAB/80  "<IMAPve_d_obj_Num>"
  Bus Selector2/74 -> ICAB/79  "<IMAPve_d_Fusion_Time_Stamp>"
  Bus Selector2/73 -> ICAB/78  "<IMAPve_d_Fusion_Status>"
  Bus Selector2/72 -> ICAB/77  "<IMAPve_d_RR_Radar_Status>"
  Bus Selector2/71 -> ICAB/76  "<IMAPve_d_LR_Radar_Status>"
  Bus Selector2/70 -> ICAB/75  "<IMAPve_d_RF_Radar_Status>"
  Bus Selector2/69 -> ICAB/74  "<IMAPve_d_Sensor_Status>"
  Bus Selector2/68 -> ICAB/73  "<IMAPve_g_ORI_R1_C2>"
  Bus Selector2/67 -> ICAB/72  "<IMAPve_g_ORI_R1_C3>"
  Bus Selector2/66 -> ICAB/71  "<IMAPve_g_ORI_R0_W>"
  Bus Selector2/65 -> ICAB/70  "<IMAPve_g_ORI_R0_VR>"
  Bus Selector2/64 -> ICAB/69  "<IMAPve_d_ORI_R0_LT>"
  Bus Selector2/63 -> ICAB/68  "<IMAPve_g_ORI_R0_C0>"
  Bus Selector2/62 -> ICAB/67  "<IMAPve_g_ORI_R0_C1>"
  Bus Selector2/61 -> ICAB/66  "<IMAPve_g_ORI_R0_C2>"
  Bus Selector2/60 -> ICAB/65  "<IMAPve_g_ORI_R0_C3>"
  Bus Selector2/59 -> ICAB/64  "<IMAPve_g_ORI_L1_W>"
  Bus Selector2/58 -> ICAB/63  "<IMAPve_g_ORI_L1_VR>"
  Bus Selector2/57 -> ICAB/62  "<IMAPve_d_ORI_L1_Type>"
  Bus Selector2/56 -> ICAB/61  "<IMAPve_g_ORI_L1_C0>"
  Bus Selector2/55 -> ICAB/60  "<IMAPve_g_ORI_L1_C1>"
  Bus Selector2/54 -> ICAB/59  "<IMAPve_g_ORI_L1_C2>"
  Bus Selector2/53 -> ICAB/58  "<IMAPve_g_ORI_L1_C3>"
  Bus Selector2/52 -> ICAB/57  "<IMAPve_g_ORI_L0_W>"
  Bus Selector2/51 -> ICAB/56  "<IMAPve_g_ORI_L0_VR>"
  Bus Selector2/50 -> ICAB/55  "<IMAPve_d_ORI_L0_Type>"
  Bus Selector2/49 -> ICAB/54  "<IMAPve_g_ORI_L0_C0>"
  Bus Selector2/48 -> ICAB/53  "<IMAPve_g_ORI_L0_C1>"
  Bus Selector2/47 -> ICAB/52  "<IMAPve_g_ORI_L0_C2>"
  Bus Selector2/46 -> ICAB/51  "<IMAPve_g_ORI_L0_C3>"
  Bus Selector2/45 -> ICAB/50  "<IMAPva_d_ORI_Obj_ID>"
  Bus Selector2/44 -> ICAB/49  "<IMAPva_g_ORI_Obj_Width>"
  Bus Selector2/43 -> ICAB/48  "<IMAPva_g_ORI_Obj_RAngle>"
  Bus Selector2/42 -> ICAB/47  "<IMAPva_g_ORI_Obj_LAngle>"
  Bus Selector2/41 -> ICAB/46  "<IMAPva_g_ORI_Obj_LongDis>"
  Bus Selector2/40 -> ICAB/45  "<IMAPve_d_ESC_Hold_State>"
  Bus Selector2/39 -> ICAB/44  "<IMAPve_d_EPB_Switch_State>"
  Bus Selector2/38 -> ICAB/43  "<IMAPve_d_EPB_Warn_Req>"
  Bus Selector2/37 -> ICAB/42  "<IMAPve_d_ACU_Passenger_Belt>"
  Bus Selector2/36 -> ICAB/41  "<IMAPve_d_BCM_BrakeLamp_State>"
  Bus Selector2/35 -> ICAB/40  "<IMAPve_d_BCM_CHMSL_Status>"
  Bus Selector2/34 -> ICAB/39  "<IMAPve_d_ESC_ACC_Active>"
  Bus Selector2/33 -> ICAB/38  "<IMAPve_d_ESC_AEB_Available>"
  Bus Selector2/32 -> ICAB/37  "<IMAPve_d_ESC_RR_Wheel_Pulse>"
  Bus Selector2/31 -> ICAB/36  "<IMAPve_d_ESC_AlarmSig>"
  Bus Selector2/30 -> ICAB/35  "<IMAPve_d_ESC_OFF>"
  Bus Selector2/29 -> ICAB/34  "<IMAPve_d_SWS_Failure_Status>"
  Bus Selector2/28 -> ICAB/33  "<IMAPve_d_BCM_Ignition_State>"
  Bus Selector2/27 -> ICAB/32  "<IMAPve_d_TCU_Actual_Gear>"
  Bus Selector2/26 -> ICAB/31  "<IMAPve_d_ESC_Veh_Standstill>"
  Bus Selector2/25 -> ICAB/30  "<IMAPve_d_EMS_AccPedal_Fault>"
  Bus Selector2/24 -> ICAB/29  "<IMAPve_g_EMS_ACC_VirtualPedal>"
  Bus Selector2/95 -> Switch3/1  "<IMAPve_d_Road_Type>"
  Bus Selector2/103 -> Switch1/1  "<IMAPve_g_L0_W>"
  Bus Selector2/111 -> Switch2/1  "<IMAPve_g_R0_W>"
  Bus Selector2/119 -> Switch/1  "<IMAPve_g_L1_W>"
  ICAB/10 -> BusCreator/10  "ICABve_g_ob7L_10"
  ICAB/9 -> BusCreator/9  "ICABve_g_ob7H_10"
  ICAB/8 -> BusCreator/8  "ICABve_g_LKATorqueReq_Value"
  ICAB/7 -> BusCreator/7  "ICABve_d_LKATorqueReq"
  ICAB/6 -> Data Type Conversion116/1, BusCreator/6, [ICABve_d_ICAState]  "ICABve_d_ICAState"
  Data Type Conversion115/1 -> BusCreator/5  "ICABve_d_ICAMode"
  ICAB/4 -> Data Type  Conversion/1
  ICAB/1 -> BusCreator/1, [ICABva_d_ICAB2ACCS]  "ICABva_d_ICAB2ACCS"
  Bus Selector3/3 -> ICAB/158  "<IMAPve_g_Camera_Signal_Fault>"
  Bus Selector3/2 -> ICAB/157  "<IMAPve_d_TSR_Sign_Type>"
  Bus Selector3/1 -> ICAB/156  "<IMAPve_d_BCM_RF_Door_State>"
  Constant6/1 -> ICAB/155
  Constant5/1 -> ICAB/154
  Constant4/1 -> ICAB/153
  Constant3/1 -> ICAB/152
  Constant2/1 -> ICAB/151
  Constant1/1 -> ICAB/150
  Constant/1 -> ICAB/149
  Data Type Conversion6/1 -> Switch/2, Switch/3
  Data Type Conversion5/1 -> Switch2/3, Switch2/2
  Data Type Conversion4/1 -> Switch1/3, Switch1/2
  Data Type Conversion3/1 -> Switch3/2, Switch3/3
  Read CM Dict2/1 -> Data Type Conversion5/1
  Compare To Constant/1 -> Enabled Subsystem/Enable
  Enabled Subsystem/1(Out1) -> Data Type Conversion45/1
  ICAB/5 -> Enabled Subsystem/1(In), Compare To Constant/1, Data Type Conversion115/1  "ICABve_d_ICAMode"
  Data Type Conversion45/1 -> Write CM Dict1/1
  Data Type  Conversion1/1 -> Write CM Dict17/1  "ICABve_g_SteerAngleCmd"
  Switch/1 -> ICAB/124  "IMAPve_g_R1_VR"
  Switch2/1 -> ICAB/116
  Switch3/1 -> ICAB/100  "L0_VR"
  Bus Selector2/143 -> ICAB/148  "<IMAPve_d_APA_AutoPark_WorkSt>"
  Switch1/1 -> ICAB/108  "IMAPve_g_R0_VR"
  Bus Selector2/23 -> ICAB/28  "<IMAPve_g_EMS_MinTWhl_Offset>"
  Bus Selector2/22 -> ICAB/27  "<IMAPve_d_PEPS_Door_Lock_Req>"
  Bus Selector2/21 -> ICAB/26  "<IMAPve_d_BCM_Trunk_State>"
  Bus Selector2/20 -> ICAB/25  "<IMAPve_g_SW_Angle_Speed>"
  Bus Selector2/19 -> ICAB/24  "<IMAPve_g_ESC_DySlope>"
  Bus Selector2/18 -> ICAB/23  "<IMAPve_g_ESC_DySlope_Accuracy>"
  Bus Selector2/17 -> ICAB/22  "<IMAPve_g_ESC_Static_Slope>"
  Bus Selector2/16 -> ICAB/21  "<IMAPve_g_ESC_Brake_Press>"
  Bus Selector2/15 -> ICAB/20  "<IMAPve_d_ESC_LonAcc_Valid>"
  Bus Selector2/14 -> ICAB/19  "<IMAPve_g_ESC_LonAcc>"
  Bus Selector2/13 -> ICAB/18  "<IMAPve_g_ESC_VehSpd>"
  Bus Selector2/12 -> ICAB/17  "<IMAPve_g_ESC_YawRate>"
  Bus Selector2/11 -> ICAB/16  "<IMAPve_d_ESC_LatAcc_Valid>"
  Bus Selector2/10 -> ICAB/15  "<IMAPve_g_ESC_LatAcc>"
  Bus Selector2/9 -> ICAB/14  "<IMAPve_d_EPS_TrqLim_State>"
  Bus Selector2/8 -> ICAB/13  "<IMAPve_d_SAS_Trim_State>"
  Bus Selector2/7 -> ICAB/12  "<IMAPve_d_SAS_Clb_State>"
  Bus Selector2/6 -> ICAB/11  "<IMAPve_d_EPS_Trq_State>"
  Bus Selector2/5 -> ICAB/10  "<IMAPve_d_EPS_LKA_State>"
  Bus Selector2/1 -> ICAB/6  "<IMAPve_d_RCTA_Swtich>"
  Bus Selector2/4 -> ICAB/9  "<IMAPve_d_JA_Alert_Switch>"
  Bus Selector2/2 -> ICAB/7  "<IMAPve_d_DOW_Switch>"
  Bus Selector2/3 -> ICAB/8  "<IMAPve_d_JA_Brake_Switch>"
  Bus Selector/2 -> ICAB/4  "<FDMMve_d_SignalTStamp>"
  ICAB/11 -> BusCreator/11  "ICABve_g_ob8H_10"
  ICAB/12 -> BusCreator/12  "ICABve_g_ob8L_10"
  ICAB/13 -> BusCreator/13  "ICABve_g_ob010H_100"
  ICAB/14 -> BusCreator/14  "ICABve_g_ob010L_100"
  ICAB/15 -> BusCreator/15  "ICABve_g_ob011H_100"
  ICAB/16 -> BusCreator/16  "ICABve_g_ob011L_100"
  ICAB/17 -> BusCreator/17  "ICABve_g_ob012H_100"
  ICAB/18 -> BusCreator/18  "ICABve_g_ob012L_100"
  Read CM Dict/1 -> Data Type Conversion6/1
  Read CM Dict1/1 -> Data Type Conversion4/1
  [EPS_LKA_State_alc] -> ICAB/5  "eps_lka_state"
  [IMAP_Output] -> Bus Selector2/1, Bus Selector3/1  "FDMM_output"
  Data Type Conversion116/1 -> Write CM Dict2/1
  Data Type  Conversion/1 -> Data Type  Conversion1/1, BusCreator/4  "ICABve_g_SteerAngleCmd"
  Read CM Dict3/1 -> Data Type Conversion3/1
  BusCreator/1 -> [ICAB_output], Bus Selector1/1
  Data Type Conversion94/1 -> ICAB/1  "System_Clock"
  ? -> ICAS_output/1, Goto1/1
  [ACCSva_d_ACCS2ICAB] -> ICAB/2  "ACCSva_d_ACCS2ICA"
  Clock/1 -> Data Type Conversion94/1
  Bus Selector/1 -> Data Type Conversion/1  "<FDMMve_d_IcaFcnConf>"
  Memory/1 -> Data Type Conversion2/1
  Bus Selector1/1 -> EPS Position Control Enable Management (EPSPCEM)_KDK1/1(EPSPCEM__bsTHmode)  "<ICABve_d_ICAMode>"
  EPS Position Control Enable Management (EPSPCEM)_KDK1/1(stEPS_State_Ctl_CMD) -> Data Type Conversion1/1  "EPS_State_Ctl"
  Data Type Conversion1/1 -> EPS_State_Mashine/1(EPS_CMD_KDK)
  EPS_State_Mashine/1(EPS_Ctr_State) -> Memory/1
  Data Type Conversion2/1 -> EPS Position Control Enable Management (EPSPCEM)_KDK1/2(EPS_Ctr_State), [EPS_LKA_State_alc]
  ICAB/2 -> BusCreator/2  "ICABve_d_SignalTStamp"
  ICAB/3 -> Demux/1, BusCreator/3  "ICABva_d_ICAB2HMI"
  [FDMM_output] -> Bus Selector/1  "FDMM_output"
  Demux/16 -> Data Type Conversion7/1
  Data Type Conversion7/1 -> Write CM Dict/1  "stLCRMode"

== system MIL4L3_SW6_V1_20220211/CarMaker/VehicleControl/Function/JA ==
  Bus Selector : BusSelector  OutputSignals=FDMMve_d_JaFcnConf
  Bus Selector1 : BusSelector  OutputSignals=IMAPve_d_JA_Alert_Switch,IMAPve_d_JA_Brake_Switch,IMAPve_g_ESC_LatAcc,IMAPve_g_ESC_YawRate,IMAPve_d_ESC_YawRate_Valid,IMAPve_g_ESC_VehSpd,IMAPve_g_ESC_LonAcc,IMAPve_d_ESC_LonAcc_Valid,IMAPve_g_ESC_Static_Slope,IMAPve_g_SW_Angle,IMAPve_g_SW_Angle_Speed,IMAPve_d_BCM_HazardLamp,IMAPve_d_BCM_Left_Light,IMAPve_d_BCM_Right_Light,IMAPve_d_BCM_Opening_State,IMAPve_g_EMS_RealPedal,IMAPve_d_ESC_Veh_Standstill,IMAPve_d_BCM_Ignition_State,IMAPve_d_ACU_Driver_Belt,IMAPve_d_SWS_Failure_Status,IMAPve_d_ESC_OFF,IMAPve_d_ESC_AlarmSig,IMAPve_d_ESC_ESC_Active,IMAPve_d_ESC_VehSpd_Valid,IMAPve_d_ESC_ABS_Active,IMAPve_d_ESC_FL_WheelPulVal,IMAPve_d_ESC_FR_WheelPulVal,IMAPve_d_ESC_RL_WheelPulVal,IMAPve_d_ESC_RR_WheelPulVal,IMAPve_d_TCU_AT_Failure,IMAPve_d_EMS_Engine_Status,IMAPve_d_ESC_AEB_Available,IMAPve_d_ESC_AEB_Active,IMAPve_d_BCM_FrontWiper_State,IMAPve_d_BCM_CHMSL_Status,IMAPve_d_BCM_BrakeLamp_State,IMAPve_d_ACU_Passenger_Belt,IMAPve_d_EMS_Brake_Pedal,IMAPve_d_EPB_Status,IMAPve_d_ESC_Drive_Direction,IMAPve_d_ESC_Hold_State,IMAPve_d_Sensor_Status,IMAPve_d_LF_Radar_Status,IMAPve_d_RF_Radar_Status,IMAPve_d_LR_Radar_Status,IMAPve_d_RR_Radar_Status,IMAPve_d_Fusion_Status,IMAPve_d_obj_Num,IMAPva_d_obj_id,IMAPva_g_obj_pos_x,IMAPva_g_obj_pos_y,IMAPva_g_obj_vel_x,IMAPva_g_obj_vel_y,IMAPva_g_obj_acc_x,IMAPva_g_obj_acc_y,IMAPva_g_obj_pos_var_x,IMAPva_g_obj_pos_var_y,IMAPva_g_obj_pos_var_xy,IMAPva_g_obj_width,IMAPva_g_obj_length,IMAPva_d_obj_class,IMAPva_d_obj_lane,IMAPva_d_obj_status,IMAPva_d_obj_age,IMAPva_d_obj_TurnLight,IMAPva_d_obj_BrakeLight,IMAPva_d_obj_MotionStatus,IMAPve_g_Camera_Signal_Fault,IMAPve_d_Camera_Status,IMAPve_d_ORI_CIPV_ID,IMAPve_d_ORI_Obj_Num,IMAPva_d_ORI_Obj_Class,IMAPva_g_ORI_Obj_RelVel,IMAPva_g_ORI_Obj_LongDis,IMAPva_g_ORI_Obj_LAngle,IMAPva_g_ORI_Obj_RAngle,IMAPva_g_ORI_Obj_Width,IMAPva_d_ORI_Obj_ID
  Bus Selector2 : BusSelector  OutputSignals=IMAPve_d_BCM_HazardLamp_Switch,IMAPve_d_ESC_MSR_Active,IMAPve_d_ESC_TCS_Active
  Bus Selector5 : BusSelector  OutputSignals=IMAPve_d_APA_AutoPark_WorkSt,IMAPve_d_EPS_Warning_State,IMAPve_d_BCM_LeftTurn_Switch,IMAPve_d_BCM_RightTurn_Switch,IMAPve_d_Radar_State,IMAPve_d_Camera_State
  Bus Selector7 : BusSelector  OutputSignals=IMAPve_d_EPS_Trq_State,IMAPve_g_EPS_SW_Trq
  BusCreator : BusCreator  Inputs=29
  Delay : Delay  DelayLength=1
  Model : ModelReference  ModelNameDialog=SW6_MIL_JABS.slxp  ModelReferenceVersion=1.495  CopyOfModelProtected=on
  tag scope: JA_output=global
  wires:
  [FDMM_output] -> Bus Selector/1
  Bus Selector/1 -> Model/1  "<FDMMve_d_JaFcnConf>"
  BusCreator/1 -> [JA_output]
  Model/1 -> BusCreator/1  "JABSve_d_Switching"
  Model/2 -> BusCreator/2  "JABSve_g_DecelReq"
  Model/3 -> BusCreator/3  "JABSve_d_FltStatus"
  Model/4 -> BusCreator/4  "JABSve_d_AlertReq"
  Model/5 -> BusCreator/5  "JABSve_d_HapticAlarm"
  Model/6 -> BusCreator/6  "JABSve_d_Tips"
  Model/7 -> BusCreator/7  "JABSve_d_DbPrefillReq"
  Model/8 -> BusCreator/8  "JABSve_d_DbFunFARCSta"
  Model/9 -> BusCreator/9  "JABSve_g_DbDecSetpoint"
  Model/10 -> BusCreator/10  "JABSve_d_DbMDDdecRequest"
  Model/11 -> BusCreator/11  "JABSve_d_DbMDDdecType"
  Model/12 -> BusCreator/12  "JABSve_d_DbHapticAlarm"
  Model/13 -> BusCreator/13  "JABSve_d_DbBraking_progress"
  Model/14 -> BusCreator/14  "JABSve_d_DbSignalTStamp"
  Model/15 -> BusCreator/15  "JABSve_d_DbJACWStatus"
  Model/16 -> BusCreator/16  "JABSve_d_DbSwitchStatus"
  Model/17 -> BusCreator/17  "JABSve_d_DbFltStatus"
  Model/18 -> BusCreator/18  "JABSve_d_DbAlertReq"
  Model/19 -> BusCreator/19  "JABSve_d_DbTips"
  Model/20 -> BusCreator/20  "JABSve_d_DbESCDriveOff"
  Model/21 -> BusCreator/21  "JABSve_d_DbESCHoldReq"
  Model/22 -> BusCreator/22  "JABSve_g_ob11H_10"
  Model/23 -> BusCreator/23  "JABSve_g_ob11L_10"
  Model/24 -> BusCreator/24  "JABSve_g_ob12H_10"
  Model/25 -> BusCreator/25  "JABSve_g_ob12L_10"
  Model/26 -> BusCreator/26  "JABSve_g_ob016H_100"
  Model/27 -> BusCreator/27  "JABSve_g_ob016L_100"
  Model/28 -> BusCreator/28  "JABSve_g_ob017H_100"
  Model/29 -> BusCreator/29  "JABSve_g_ob017L_100"
  [MDD_deceleration_type] -> Model/80  "ADAS_deceleration_type"
  [IMAP_Output] -> Bus Selector1/1, Bus Selector2/1, Bus Selector7/1, Bus Selector5/1
  [ADAS_AEBAlertReq] -> Delay/1
  Bus Selector1/7 -> Model/8  "<IMAPve_g_ESC_LonAcc>"
  Bus Selector1/8 -> Model/9  "<IMAPve_d_ESC_LonAcc_Valid>"
  Bus Selector1/6 -> Model/7  "<IMAPve_g_ESC_VehSpd>"
  Bus Selector1/9 -> Model/10  "<IMAPve_g_ESC_Static_Slope>"
  Bus Selector1/5 -> Model/6  "<IMAPve_d_ESC_YawRate_Valid>"
  Bus Selector1/10 -> Model/11  "<IMAPve_g_SW_Angle>"
  Bus Selector1/4 -> Model/5  "<IMAPve_g_ESC_YawRate>"
  Bus Selector1/11 -> Model/12  "<IMAPve_g_SW_Angle_Speed>"
  Bus Selector1/3 -> Model/4  "<IMAPve_g_ESC_LatAcc>"
  Bus Selector1/12 -> Model/13  "<IMAPve_d_BCM_HazardLamp>"
  Bus Selector1/2 -> Model/3  "<IMAPve_d_JA_Brake_Switch>"
  Bus Selector1/13 -> Model/14  "<IMAPve_d_BCM_Left_Light>"
  Bus Selector1/1 -> Model/2  "<IMAPve_d_JA_Alert_Switch>"
  Bus Selector1/14 -> Model/15  "<IMAPve_d_BCM_Right_Light>"
  Bus Selector1/15 -> Model/16  "<IMAPve_d_BCM_Opening_State>"
  Bus Selector1/16 -> Model/17  "<IMAPve_g_EMS_RealPedal>"
  Bus Selector1/17 -> Model/18  "<IMAPve_d_ESC_Veh_Standstill>"
  Bus Selector1/18 -> Model/19  "<IMAPve_d_BCM_Ignition_State>"
  Bus Selector1/19 -> Model/20  "<IMAPve_d_ACU_Driver_Belt>"
  Bus Selector1/20 -> Model/21  "<IMAPve_d_SWS_Failure_Status>"
  Bus Selector1/21 -> Model/22  "<IMAPve_d_ESC_OFF>"
  Bus Selector1/22 -> Model/23  "<IMAPve_d_ESC_AlarmSig>"
  Bus Selector1/23 -> Model/24  "<IMAPve_d_ESC_ESC_Active>"
  Bus Selector1/24 -> Model/25  "<IMAPve_d_ESC_VehSpd_Valid>"
  Bus Selector1/25 -> Model/26  "<IMAPve_d_ESC_ABS_Active>"
  Bus Selector1/26 -> Model/27  "<IMAPve_d_ESC_FL_WheelPulVal>"
  Bus Selector1/27 -> Model/28  "<IMAPve_d_ESC_FR_WheelPulVal>"
  Bus Selector1/28 -> Model/29  "<IMAPve_d_ESC_RL_WheelPulVal>"
  Bus Selector1/29 -> Model/30  "<IMAPve_d_ESC_RR_WheelPulVal>"
  Bus Selector1/30 -> Model/31  "<IMAPve_d_TCU_AT_Failure>"
  Bus Selector1/31 -> Model/32  "<IMAPve_d_EMS_Engine_Status>"
  Bus Selector1/32 -> Model/33  "<IMAPve_d_ESC_AEB_Available>"
  Bus Selector1/33 -> Model/34  "<IMAPve_d_ESC_AEB_Active>"
  Bus Selector1/34 -> Model/35  "<IMAPve_d_BCM_FrontWiper_State>"
  Bus Selector1/35 -> Model/36  "<IMAPve_d_BCM_CHMSL_Status>"
  Bus Selector1/36 -> Model/37  "<IMAPve_d_BCM_BrakeLamp_State>"
  Bus Selector1/37 -> Model/38  "<IMAPve_d_ACU_Passenger_Belt>"
  Bus Selector1/38 -> Model/39  "<IMAPve_d_EMS_Brake_Pedal>"
  Bus Selector1/39 -> Model/40  "<IMAPve_d_EPB_Status>"
  Bus Selector1/40 -> Model/41  "<IMAPve_d_ESC_Drive_Direction>"
  Bus Selector1/41 -> Model/42  "<IMAPve_d_ESC_Hold_State>"
  Bus Selector1/42 -> Model/43  "<IMAPve_d_Sensor_Status>"
  Bus Selector1/43 -> Model/44  "<IMAPve_d_LF_Radar_Status>"
  Bus Selector1/44 -> Model/45  "<IMAPve_d_RF_Radar_Status>"
  Bus Selector1/45 -> Model/46  "<IMAPve_d_LR_Radar_Status>"
  Bus Selector1/46 -> Model/47  "<IMAPve_d_RR_Radar_Status>"
  Bus Selector1/47 -> Model/48  "<IMAPve_d_Fusion_Status>"
  Bus Selector1/48 -> Model/49  "<IMAPve_d_obj_Num>"
  Bus Selector1/49 -> Model/50  "<IMAPva_d_obj_id>"
  Bus Selector1/50 -> Model/51  "<IMAPva_g_obj_pos_x>"
  Bus Selector1/51 -> Model/52  "<IMAPva_g_obj_pos_y>"
  Bus Selector1/52 -> Model/53  "<IMAPva_g_obj_vel_x>"
  Bus Selector1/53 -> Model/54  "<IMAPva_g_obj_vel_y>"
  Bus Selector1/54 -> Model/55  "<IMAPva_g_obj_acc_x>"
  Bus Selector1/55 -> Model/56  "<IMAPva_g_obj_acc_y>"
  Bus Selector1/56 -> Model/57  "<IMAPva_g_obj_pos_var_x>"
  Bus Selector1/57 -> Model/58  "<IMAPva_g_obj_pos_var_y>"
  Bus Selector1/58 -> Model/59  "<IMAPva_g_obj_pos_var_xy>"
  Bus Selector1/59 -> Model/60  "<IMAPva_g_obj_width>"
  Bus Selector1/60 -> Model/61  "<IMAPva_g_obj_length>"
  Bus Selector1/61 -> Model/62  "<IMAPva_d_obj_class>"
  Bus Selector1/62 -> Model/63  "<IMAPva_d_obj_lane>"
  Bus Selector1/63 -> Model/64  "<IMAPva_d_obj_status>"
  Bus Selector1/64 -> Model/65  "<IMAPva_d_obj_age>"
  Bus Selector1/65 -> Model/66  "<IMAPva_d_obj_TurnLight>"
  Bus Selector1/66 -> Model/67  "<IMAPva_d_obj_BrakeLight>"
  Bus Selector1/67 -> Model/68  "<IMAPva_d_obj_MotionStatus>"
  Bus Selector1/68 -> Model/69  "<IMAPve_g_Camera_Signal_Fault>"
  Bus Selector1/69 -> Model/70  "<IMAPve_d_Camera_Status>"
  Bus Selector1/70 -> Model/71  "<IMAPve_d_ORI_CIPV_ID>"
  Bus Selector1/71 -> Model/72  "<IMAPve_d_ORI_Obj_Num>"
  Bus Selector1/72 -> Model/73  "<IMAPva_d_ORI_Obj_Class>"
  Bus Selector1/73 -> Model/74  "<IMAPva_g_ORI_Obj_RelVel>"
  Bus Selector1/74 -> Model/75  "<IMAPva_g_ORI_Obj_LongDis>"
  Bus Selector1/75 -> Model/76  "<IMAPva_g_ORI_Obj_LAngle>"
  Bus Selector1/76 -> Model/77  "<IMAPva_g_ORI_Obj_RAngle>"
  Bus Selector1/77 -> Model/78  "<IMAPva_g_ORI_Obj_Width>"
  Bus Selector1/78 -> Model/79  "<IMAPva_d_ORI_Obj_ID>"
  Bus Selector5/2 -> Model/82  "<IMAPve_d_EPS_Warning_State>"
  Bus Selector5/1 -> Model/81  "<IMAPve_d_APA_AutoPark_WorkSt>"
  Bus Selector5/3 -> Model/83  "<IMAPve_d_BCM_LeftTurn_Switch>"
  Bus Selector5/4 -> Model/84  "<IMAPve_d_BCM_RightTurn_Switch>"
  Bus Selector5/5 -> Model/85  "<IMAPve_d_Radar_State>"
  Bus Selector5/6 -> Model/86  "<IMAPve_d_Camera_State>"
  Bus Selector7/1 -> Model/88  "<IMAPve_d_EPS_Trq_State>"
  Bus Selector7/2 -> Model/89  "<IMAPve_g_EPS_SW_Trq>"
  Bus Selector2/1 -> Model/93  "<IMAPve_d_BCM_HazardLamp_Switch>"
  Bus Selector2/2 -> Model/94  "<IMAPve_d_ESC_MSR_Active>"
  Bus Selector2/3 -> Model/95  "<IMAPve_d_ESC_TCS_Active>"
  Delay/1 -> Model/87
